simulink model "full_car_state_space_model"  (Simulink 8.2)
settings: Solver=ode45  StartTime=0.0  StopTime=10.0  RelTol=1e-3
values from neighbouring files (symbols this model uses):
  Ao = [zeros(7) eye(7) ... (first row only)    [car_sis.m]
  Bo = [zeros(8,4) ... (first row only)    [car_sis.m]
  CCo = [1 0 0 0 0 0 0 0 0 0 0 0 0 0]    [car_sis.m]
  Do = zeros(1,4)    [car_sis.m]
  Lo1 = 1.2    [car_sis.m]
  Lo2 = 1.    (= 1)    [car_sis.m]
  Vo = 50    [car.m]    (also in car_sis.m = 16.6666666667)
settings Model: Creator=DOAN  LastModifiedBy=oguzhan
settings DataIOCC: SignalLoggingSaveFormat=Dataset
settings OptimizationCC: ExpressionDepthLimit=128
settings DebuggingCC: FcnCallInpInsideContextMsg=EnableAllAsError  StateNameClashWarn=none
settings GRTTargetCC: CombineOutputUpdateFcns=on  GRTInterface=off

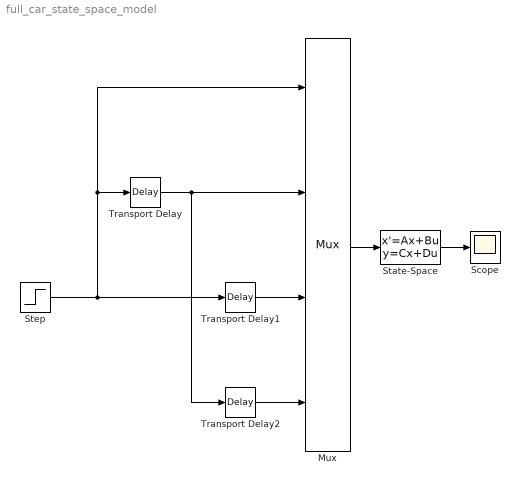
== system full_car_state_space_model ==
  Mux : Mux
  Scope : Scope
  State-Space : StateSpace  A=Ao  B=Bo  C=CCo  D=Do  X0=0
  Step : Step  SampleTime=0
  Transport Delay : TransportDelay  DelayTime=(Lo1+Lo2)/Vo
  Transport Delay1 : TransportDelay  DelayTime=0.001
  Transport Delay2 : TransportDelay  DelayTime=0.001
  wires:
  Mux/1 -> State-Space/1
  Step/1 -> Mux/1, Transport Delay/1, Transport Delay1/1
  State-Space/1 -> Scope/1
  Transport Delay/1 -> Mux/2, Transport Delay2/1
  Transport Delay1/1 -> Mux/3
  Transport Delay2/1 -> Mux/4
